simulink library "Pitch_on_Roll__Lib"  (R2024b)
settings: Solver=VariableStepAuto  StartTime=0.0  StopTime=10.0  RelTol=1e-3
undefined symbols (not defined in the file or in its folder): axisCmdType, baseAccEcho, baseRatesEcho, cmdTypes, Motion, Support
libraries: nesl_utility x34, fl_lib x18, sm_lib x4, simulink_extras x1
(part 2 of 2)

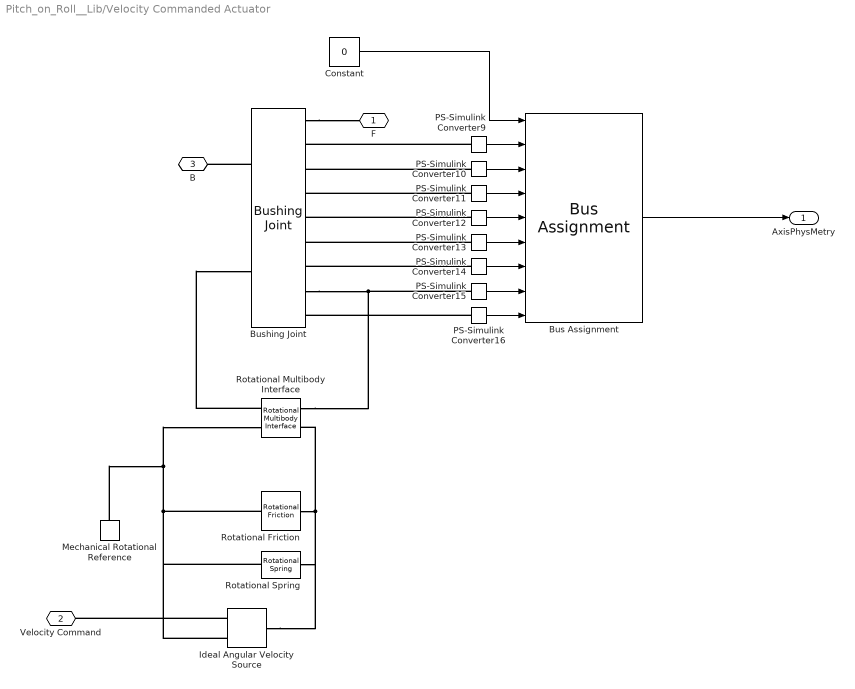
== system Pitch_on_Roll__Lib/Velocity Commanded Actuator ==
  Bus Assignment : BusAssignment  AssignedSignals=Support.pX,Support.pY,Support.pZ,Support.qX,Support.qY,Motion.AxisPosition,Motion.AxisVelocity,Motion.AxisTorque
  Bushing Joint : sm_lib/Joints/Bushing Joint  JointMode=Normal  CompositeWrenchDir=FollowerOnBase  CompositeWrenchFrame=BaseFrame  SenseConstraintForce=off  SenseConstraintTorque=off  SenseTotalForce=off  SenseTotalTorque=off  PxPositionTargetSpecify=off  PxPositionTargetPriority=High  PxPositionTargetValue=0  PxPositionTargetValueUnits=m  PxVelocityTargetSpecify=off  PxVelocityTargetPriority=High  PxVelocityTargetValue=0  PxVelocityTargetValueUnits=m/s  PxEquilibriumPosition=0.0  PxEquilibriumPositionUnits=mm  PxSpringStiffness=bearingProps.Krad  PxSpringStiffnessUnits=N/mm  PxDampingCoefficient=bearingProps.Crad  PxDampingCoefficientUnits=N/(m/s)  PxLowerLimitSpecify=off  PxLowerLimitBound=-1  PxLowerLimitBoundUnits=m  PxLowerLimitStiffness=1e6  PxLowerLimitStiffnessUnits=N/m  PxLowerLimitDamping=1e3  PxLowerLimitDampingUnits=N/(m/s)  PxLowerLimitTransitionRegionWidth=1e-4  PxLowerLimitTransitionRegionWidthUnits=m  PxUpperLimitSpecify=off  PxUpperLimitBound=1  PxUpperLimitBoundUnits=m  PxUpperLimitStiffness=1e6  PxUpperLimitStiffnessUnits=N/m  PxUpperLimitDamping=1e3  PxUpperLimitDampingUnits=N/(m/s)  PxUpperLimitTransitionRegionWidth=1e-4  PxUpperLimitTransitionRegionWidthUnits=m  PxTorqueActuationMode=NoTorque  PxMotionActuationMode=ComputedMotion  PxSensePosition=on  PxSenseVelocity=off  PxSenseAcceleration=off  PxSenseTorqueForce=off  PxSenseLowerLimitTorqueForce=off  PxSenseUpperLimitTorqueForce=off  PyPositionTargetSpecify=off  PyPositionTargetPriority=High  PyPositionTargetValue=0  PyPositionTargetValueUnits=m  PyVelocityTargetSpecify=off  PyVelocityTargetPriority=High  PyVelocityTargetValue=0  PyVelocityTargetValueUnits=m/s  PyEquilibriumPosition=0  PyEquilibriumPositionUnits=m  PySpringStiffness=bearingProps.Krad  PySpringStiffnessUnits=N/mm  PyDampingCoefficient=bearingProps.Crad  PyDampingCoefficientUnits=N/(m/s)  PyLowerLimitSpecify=off  PyLowerLimitBound=-1  PyLowerLimitBoundUnits=m  PyLowerLimitStiffness=1e6  PyLowerLimitStiffnessUnits=N/m  PyLowerLimitDamping=1e3  PyLowerLimitDampingUnits=N/(m/s)  PyLowerLimitTransitionRegionWidth=1e-4  PyLowerLimitTransitionRegionWidthUnits=m  PyUpperLimitSpecify=off  PyUpperLimitBound=1  PyUpperLimitBoundUnits=m  PyUpperLimitStiffness=1e6  PyUpperLimitStiffnessUnits=N/m  PyUpperLimitDamping=1e3  PyUpperLimitDampingUnits=N/(m/s)  PyUpperLimitTransitionRegionWidth=1e-4  PyUpperLimitTransitionRegionWidthUnits=m  PyTorqueActuationMode=NoTorque  PyMotionActuationMode=ComputedMotion  PySensePosition=on  PySenseVelocity=off  PySenseAcceleration=off  PySenseTorqueForce=off  PySenseLowerLimitTorqueForce=off  PySenseUpperLimitTorqueForce=off  PzPositionTargetSpecify=off  PzPositionTargetPriority=High  PzPositionTargetValue=0  PzPositionTargetValueUnits=m  PzVelocityTargetSpecify=off  PzVelocityTargetPriority=High  PzVelocityTargetValue=0  PzVelocityTargetValueUnits=m/s  PzEquilibriumPosition=0.0  PzEquilibriumPositionUnits=mm  PzSpringStiffness=bearingProps.Kax  PzSpringStiffnessUnits=N/mm  PzDampingCoefficient=bearingProps.Cax  PzDampingCoefficientUnits=N/(m/s)  PzLowerLimitSpecify=off  PzLowerLimitBound=-1  PzLowerLimitBoundUnits=m  PzLowerLimitStiffness=1e6  PzLowerLimitStiffnessUnits=N/m  PzLowerLimitDamping=1e3  PzLowerLimitDampingUnits=N/(m/s)  PzLowerLimitTransitionRegionWidth=1e-4  PzLowerLimitTransitionRegionWidthUnits=m  PzUpperLimitSpecify=off  PzUpperLimitBound=1  PzUpperLimitBoundUnits=m  PzUpperLimitStiffness=1e6  PzUpperLimitStiffnessUnits=N/m  PzUpperLimitDamping=1e3  PzUpperLimitDampingUnits=N/(m/s)  PzUpperLimitTransitionRegionWidth=1e-4  PzUpperLimitTransitionRegionWidthUnits=m  PzTorqueActuationMode=NoTorque  PzMotionActuationMode=ComputedMotion  PzSensePosition=on  PzSenseVelocity=off  PzSenseAcceleration=off  PzSenseTorqueForce=off  PzSenseLowerLimitTorqueForce=off  PzSenseUpperLimitTorqueForce=off  RxPositionTargetSpecify=off  RxPositionTargetPriority=High  RxPositionTargetValue=0  RxPositionTargetValueUnits=deg  RxVelocityTargetSpecify=off  RxVelocityTargetPriority=High  RxVelocityTargetValue=0  RxVelocityTargetValueUnits=deg/s  RxEquilibriumPosition=0.0  RxEquilibriumPositionUnits=deg  RxSpringStiffness=bearingProps.Kang  RxSpringStiffnessUnits=N*m/rad  RxDampingCoefficient=bearingProps.Cang  RxDampingCoefficientUnits=N*m*s/rad  RxLowerLimitSpecify=off  RxLowerLimitBound=-90  RxLowerLimitBoundUnits=deg  RxLowerLimitStiffness=1e4  RxLowerLimitStiffnessUnits=N*m/deg  RxLowerLimitDamping=10  RxLowerLimitDampingUnits=N*m/(deg/s)  RxLowerLimitTransitionRegionWidth=0.1  RxLowerLimitTransitionRegionWidthUnits=deg  RxUpperLimitSpecify=off  RxUpperLimitBound=90  RxUpperLimitBoundUnits=deg  RxUpperLimitStiffness=1e4  RxUpperLimitStiffnessUnits=N*m/deg  RxUpperLimitDamping=10  RxUpperLimitDampingUnits=N*m/(deg/s)  RxUpperLimitTransitionRegionWidth=0.1  RxUpperLimitTransitionRegionWidthUnits=deg  RxTorqueActuationMode=NoTorque  RxMotionActuationMode=ComputedMotion  RxSensePosition=on  RxSenseVelocity=off  RxSenseAcceleration=off  RxSenseTorqueForce=off  RxSenseLowerLimitTorqueForce=off  RxSenseUpperLimitTorqueForce=off  RyPositionTargetSpecify=off  RyPositionTargetPriority=High  RyPositionTargetValue=0  RyPositionTargetValueUnits=deg  RyVelocityTargetSpecify=off  RyVelocityTargetPriority=High  RyVelocityTargetValue=0  RyVelocityTargetValueUnits=deg/s  RyEquilibriumPosition=0.0  RyEquilibriumPositionUnits=deg  RySpringStiffness=bearingProps.Kang  RySpringStiffnessUnits=N*m/rad  RyDampingCoefficient=bearingProps.Cang  RyDampingCoefficientUnits=N*m*s/rad  RyLowerLimitSpecify=off  RyLowerLimitBound=-90  RyLowerLimitBoundUnits=deg  RyLowerLimitStiffness=1e4  RyLowerLimitStiffnessUnits=N*m/deg  RyLowerLimitDamping=10  RyLowerLimitDampingUnits=N*m/(deg/s)  RyLowerLimitTransitionRegionWidth=0.1  RyLowerLimitTransitionRegionWidthUnits=deg  RyUpperLimitSpecify=off  RyUpperLimitBound=90  RyUpperLimitBoundUnits=deg  RyUpperLimitStiffness=1e4  RyUpperLimitStiffnessUnits=N*m/deg  RyUpperLimitDamping=10  RyUpperLimitDampingUnits=N*m/(deg/s)  RyUpperLimitTransitionRegionWidth=0.1  RyUpperLimitTransitionRegionWidthUnits=deg  RyTorqueActuationMode=NoTorque  RyMotionActuationMode=ComputedMotion  RySensePosition=on  RySenseVelocity=off  RySenseAcceleration=off  RySenseTorqueForce=off  RySenseLowerLimitTorqueForce=off  RySenseUpperLimitTorqueForce=off  RzPositionTargetSpecify=off  RzPositionTargetPriority=High  RzPositionTargetValue=0  RzPositionTargetValueUnits=deg  RzVelocityTargetSpecify=off  RzVelocityTargetPriority=High  RzVelocityTargetValue=0  RzVelocityTargetValueUnits=deg/s  RzEquilibriumPosition=0  RzEquilibriumPositionUnits=deg  RzSpringStiffness=0  RzSpringStiffnessUnits=N*m/deg  RzDampingCoefficient=0  RzDampingCoefficientUnits=N*m/(deg/s)  RzLowerLimitSpecify=off  RzLowerLimitBound=-90  RzLowerLimitBoundUnits=deg  RzLowerLimitStiffness=1e4  RzLowerLimitStiffnessUnits=N*m/deg  RzLowerLimitDamping=10  RzLowerLimitDampingUnits=N*m/(deg/s)  RzLowerLimitTransitionRegionWidth=0.1  RzLowerLimitTransitionRegionWidthUnits=deg  RzUpperLimitSpecify=off  RzUpperLimitBound=90  RzUpperLimitBoundUnits=deg  RzUpperLimitStiffness=1e4  RzUpperLimitStiffnessUnits=N*m/deg  RzUpperLimitDamping=10  RzUpperLimitDampingUnits=N*m/(deg/s)  RzUpperLimitTransitionRegionWidth=0.1  RzUpperLimitTransitionRegionWidthUnits=deg  RzTorqueActuationMode=InputTorque  RzMotionActuationMode=ComputedMotion  RzSensePosition=on  RzSenseVelocity=on  RzSenseAcceleration=off  RzSenseTorqueForce=on  RzSenseLowerLimitTorqueForce=off  RzSenseUpperLimitTorqueForce=off
  Constant : Constant  Value=0  OutDataTypeStr=Bus: AxisMetry
  Ideal Angular Velocity Source : fl_lib/Mechanical/Mechanical Sources/Ideal Angular Velocity Source
  Mechanical Rotational Reference : fl_lib/Mechanical/Rotational Elements/Mechanical Rotational Reference
  PS-Simulink Converter10 : nesl_utility/PS-Simulink Converter  PhysicalDomain=network_engine_domain  SubClassName=ps_output  LeftPortType=input  RightPortType=output  PseudoPeriodic=off  Frequencies=[]  VectorFormat=inherit  Unit=m  AffineConversion=off
  PS-Simulink Converter11 : nesl_utility/PS-Simulink Converter  PhysicalDomain=network_engine_domain  SubClassName=ps_output  LeftPortType=input  RightPortType=output  PseudoPeriodic=off  Frequencies=[]  VectorFormat=inherit  Unit=m  AffineConversion=off
  PS-Simulink Converter12 : nesl_utility/PS-Simulink Converter  PhysicalDomain=network_engine_domain  SubClassName=ps_output  LeftPortType=input  RightPortType=output  PseudoPeriodic=off  Frequencies=[]  VectorFormat=inherit  Unit=rad  AffineConversion=off
  PS-Simulink Converter13 : nesl_utility/PS-Simulink Converter  PhysicalDomain=network_engine_domain  SubClassName=ps_output  LeftPortType=input  RightPortType=output  PseudoPeriodic=off  Frequencies=[]  VectorFormat=inherit  Unit=rad  AffineConversion=off
  PS-Simulink Converter14 : nesl_utility/PS-Simulink Converter  PhysicalDomain=network_engine_domain  SubClassName=ps_output  LeftPortType=input  RightPortType=output  PseudoPeriodic=off  Frequencies=[]  VectorFormat=inherit  Unit=rad  AffineConversion=off
  PS-Simulink Converter15 : nesl_utility/PS-Simulink Converter  PhysicalDomain=network_engine_domain  SubClassName=ps_output  LeftPortType=input  RightPortType=output  PseudoPeriodic=off  Frequencies=[]  VectorFormat=inherit  Unit=rad/s  AffineConversion=off
  PS-Simulink Converter16 : nesl_utility/PS-Simulink Converter  PhysicalDomain=network_engine_domain  SubClassName=ps_output  LeftPortType=input  RightPortType=output  PseudoPeriodic=off  Frequencies=[]  VectorFormat=inherit  Unit=N*m  AffineConversion=off
  PS-Simulink Converter9 : nesl_utility/PS-Simulink Converter  PhysicalDomain=network_engine_domain  SubClassName=ps_output  LeftPortType=input  RightPortType=output  PseudoPeriodic=off  Frequencies=[]  VectorFormat=inherit  Unit=m  AffineConversion=off
  Rotational Friction : fl_lib/Mechanical/Rotational Elements/Rotational Friction  brkwy_trq=bearingProps.Tf*1.4 m*mN  brkwy_vel=0.1 rad/s  Col_trq=bearingProps.Tf m*mN  visc_coef=0.0 N*m*s/rad  w_specify=off  w_priority=None  w=0 rad/s  w_nominal_specify=off  w_nominal_value=1  w_nominal_unit=rad/s  t_specify=off  t_priority=None  t=0 N*m  t_nominal_specify=off  t_nominal_value=1  t_nominal_unit=N*m
  Rotational Multibody Interface : fl_lib/Mechanical/Multibody Interfaces/Rotational Multibody Interface
  Rotational Spring : fl_lib/Mechanical/Rotational Elements/Rotational Spring  spr_rate=harnessConstant m*mN/rad  w_specify=off  w_priority=None  w=0 rad/s  w_nominal_specify=off  w_nominal_value=1  w_nominal_unit=rad/s  t_specify=off  t_priority=None  t=0 N*m  t_nominal_specify=off  t_nominal_value=1  t_nominal_unit=N*m  phi_specify=off  phi_priority=High  phi=0 rad  phi_nominal_specify=off  phi_nominal_value=1  phi_nominal_unit=rad
  F : PMIOPort  Side=Right
  Velocity Command : PMIOPort  Port=2  Side=Left
  B : PMIOPort  Port=3  Side=Left
  AxisPhysMetry : Outport
  wires:
  Constant/1 -> Bus Assignment/1
  Bus Assignment/1 -> AxisPhysMetry/1
  PS-Simulink Converter11/1 -> Bus Assignment/4
  PS-Simulink Converter12/1 -> Bus Assignment/5
  PS-Simulink Converter14/1 -> Bus Assignment/7
  PS-Simulink Converter13/1 -> Bus Assignment/6
  PS-Simulink Converter15/1 -> Bus Assignment/8
  PS-Simulink Converter10/1 -> Bus Assignment/3
  PS-Simulink Converter16/1 -> Bus Assignment/9
  PS-Simulink Converter9/1 -> Bus Assignment/2
  connections:
  Ideal Angular Velocity Source/RConn2 -- Rotational Spring/RConn1 -- Rotational Friction/RConn1 -- Mechanical Rotational Reference/LConn1 -- Rotational Multibody Interface/LConn2
  PS-Simulink Converter16/LConn1 -- Bushing Joint/RConn9
  Rotational Multibody Interface/LConn1 -- Bushing Joint/LConn2
  Ideal Angular Velocity Source/LConn1 -- Rotational Spring/LConn1 -- Rotational Multibody Interface/RConn2 -- Rotational Friction/LConn1
  PS-Simulink Converter13/LConn1 -- Bushing Joint/RConn6
  PS-Simulink Converter11/LConn1 -- Bushing Joint/RConn4
  PS-Simulink Converter12/LConn1 -- Bushing Joint/RConn5
  Rotational Multibody Interface/RConn1 -- PS-Simulink Converter15/LConn1 -- Bushing Joint/RConn8
  PS-Simulink Converter9/LConn1 -- Bushing Joint/RConn2
  PS-Simulink Converter14/LConn1 -- Bushing Joint/RConn7
  Bushing Joint/RConn1 -- F/RConn1
  Bushing Joint/LConn1 -- B/RConn1
  PS-Simulink Converter10/LConn1 -- Bushing Joint/RConn3
  Ideal Angular Velocity Source/RConn1 -- Velocity Command/RConn1

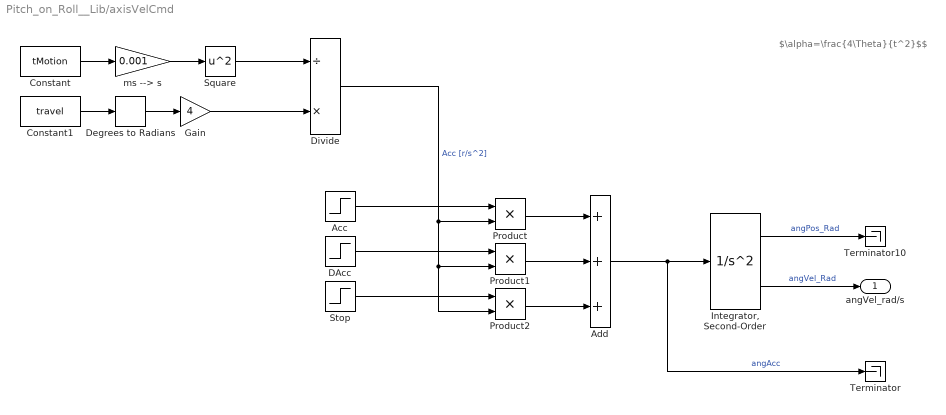
== system Pitch_on_Roll__Lib/axisVelCmd ==
  note: $\alpha=\frac{4\Theta}{t^2}$$
  Acc : Step  Time=tStart  SampleTime=0
  Add : Sum  Inputs=3
  Constant : Constant  Value=tMotion
  Constant1 : Constant  Value=travel
  DAcc : Step  Time=tStart+tMotion/2000  After=-2  SampleTime=0
  Degrees to Radians : simulink_extras/Transformations/Degrees to Radians
  Divide : Product  Inputs=/*
  Gain : Gain  Gain=4
  "Integrator, Second-Order" : SecondOrderIntegrator
  Product : Product
  Product1 : Product
  Product2 : Product
  Square : Math  Operator=square
  Stop : Step  Time=tStart+tMotion/1000  SampleTime=0
  Terminator : Terminator
  Terminator10 : Terminator
  ms --> s : Gain  Gain=0.001
  angVel_rad/s : Outport
  wires:
  Add/1 -> Terminator/1, "Integrator, Second-Order"/1  "angAcc"
  Stop/1 -> Product2/1
  "Integrator, Second-Order"/1 -> Terminator10/1  "angPos_Rad"
  Acc/1 -> Product/1
  DAcc/1 -> Product1/1
  "Integrator, Second-Order"/2 -> angVel_rad/s/1  "angVel_Rad"
  Constant1/1 -> Degrees to Radians/1
  Degrees to Radians/1 -> Gain/1
  Constant/1 -> ms --> s/1
  ms --> s/1 -> Square/1
  Gain/1 -> Divide/2
  Square/1 -> Divide/1
  Divide/1 -> Product/2, Product1/2, Product2/2  "Acc [r/s^2]"
  Product/1 -> Add/1
  Product1/1 -> Add/2
  Product2/1 -> Add/3

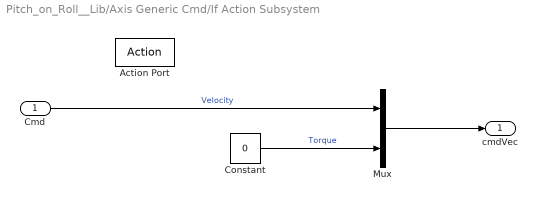
== system Pitch_on_Roll__Lib/Axis Generic Cmd/If Action Subsystem ==
  Cmd : Inport
  Action Port : ActionPort
  Constant : Constant  Value=0
  Mux : Mux  Inputs=2
  cmdVec : Outport
  wires:
  Cmd/1 -> Mux/1  "Velocity"
  Constant/1 -> Mux/2  "Torque"
  Mux/1 -> cmdVec/1

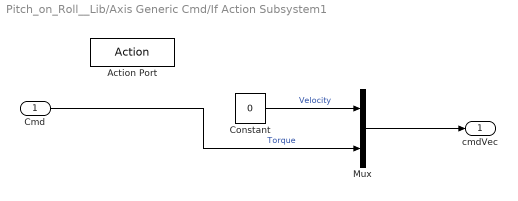
== system Pitch_on_Roll__Lib/Axis Generic Cmd/If Action Subsystem1 ==
  Cmd : Inport
  Action Port : ActionPort
  Constant : Constant  Value=0
  Mux : Mux  Inputs=2
  cmdVec : Outport
  wires:
  Mux/1 -> cmdVec/1
  Cmd/1 -> Mux/2  "Torque"
  Constant/1 -> Mux/1  "Velocity"

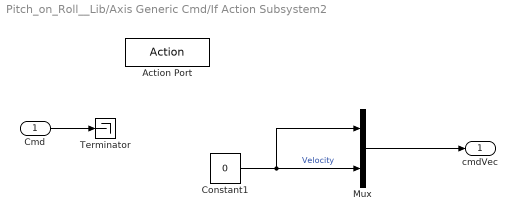
== system Pitch_on_Roll__Lib/Axis Generic Cmd/If Action Subsystem2 ==
  Cmd : Inport
  Action Port : ActionPort
  Constant1 : Constant  Value=0
  Mux : Mux  Inputs=2
  Terminator : Terminator
  cmdVec : Outport
  wires:
  Cmd/1 -> Terminator/1
  Mux/1 -> cmdVec/1
  Constant1/1 -> Mux/1, Mux/2  "Velocity"

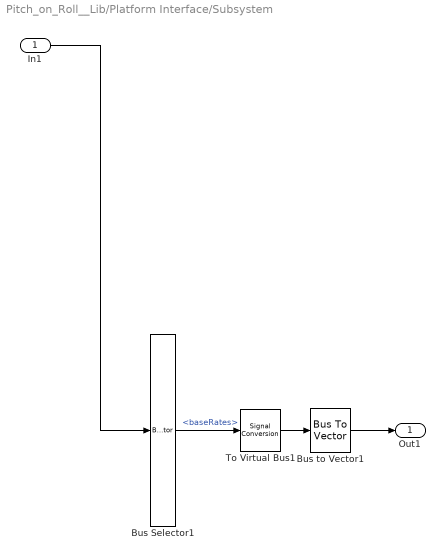
== system Pitch_on_Roll__Lib/Platform Interface/Subsystem ==
  In1 : Inport
  Bus Selector1 : BusSelector  OutputSignals=baseRates
  Bus to Vector1 : BusToVector
  To Virtual Bus1 : SignalConversion  ConversionOutput=Virtual bus  OverrideOpt=off
  Out1 : Outport
  wires:
  Bus Selector1/1 -> To Virtual Bus1/1  "<baseRates>"
  To Virtual Bus1/1 -> Bus to Vector1/1
  Bus to Vector1/1 -> Out1/1
  In1/1 -> Bus Selector1/1
